simulink library "linearization"  (R2016b)
settings: Solver=VariableStepAuto  StartTime=0.0  StopTime=10.0  RelTol=1e-3
undefined symbols (not defined in the file): fsw_params
libraries: aerolibutil x2, simulink_extras x1
settings Model: Creator=bijan  LastModifiedBy=bijan

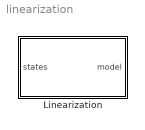
== system linearization ==
  Linearization : Subsystem

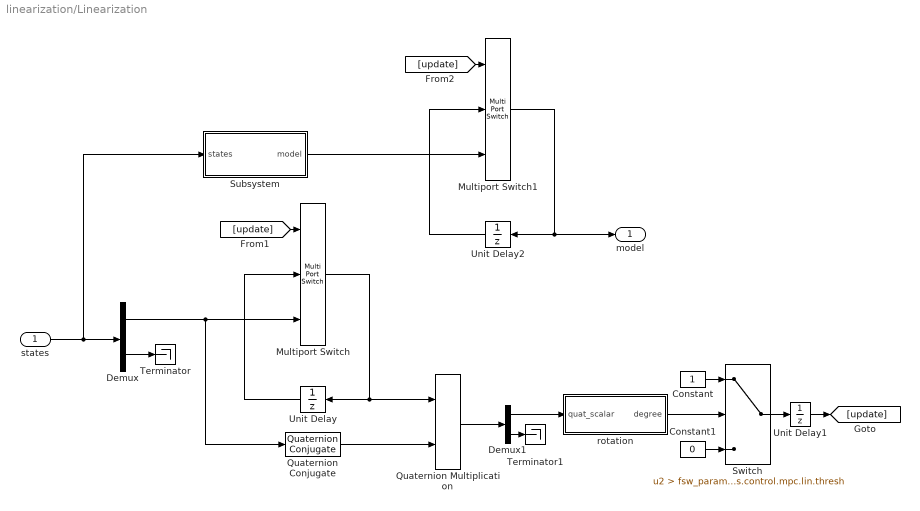
== system linearization/Linearization ==
  states : Inport
  Constant : Constant
  Constant1 : Constant  Value=0
  Demux : Demux  Outputs=[4 3]
  Demux1 : Demux  Outputs=[1 3]
  Multiport Switch : MultiPortSwitch  DataPortOrder=Zero-based contiguous  Inputs=2  DataPortIndices={0,1}
  Multiport Switch1 : MultiPortSwitch  DataPortOrder=Zero-based contiguous  Inputs=2  DataPortIndices={0,1}
  Quaternion Conjugate : aerolibutil/Quaternion Conjugate
  Quaternion Multiplication : aerolibutil/Quaternion Multiplication
  Subsystem : Subsystem
  Switch : Switch  Criteria=u2 > Threshold  Threshold=fsw_params.control.mpc.lin.thresh
  Terminator : Terminator
  Terminator1 : Terminator
  Unit Delay : UnitDelay  InitialCondition=fsw_params.control.mpc.lin.ic_quat_ud  SampleTime=-1
  Unit Delay1 : UnitDelay  InitialCondition=fsw_params.control.mpc.lin.ic_update_ud  SampleTime=-1
  Unit Delay2 : UnitDelay  InitialCondition=fsw_params.control.mpc.lin.bus_ic  SampleTime=-1
  rotation : Subsystem
  model : Outport
  wires:
  states/1 -> Subsystem/1(states), Demux/1
  Demux/2 -> Terminator/1
  Demux/1 -> Quaternion Conjugate/1, Multiport Switch/3
  Multiport Switch/1 -> Unit Delay/1, Quaternion Multiplication/1
  Unit Delay/1 -> Multiport Switch/2
  Quaternion Conjugate/1 -> Quaternion Multiplication/2
  Quaternion Multiplication/1 -> Demux1/1
  Demux1/2 -> Terminator1/1
  Demux1/1 -> rotation/1(quat_scalar)
  rotation/1(degree) -> Switch/2
  Constant/1 -> Switch/1
  Constant1/1 -> Switch/3
  Switch/1 -> Unit Delay1/1
  [update] -> Multiport Switch/1
  Unit Delay1/1 -> [update]
  Unit Delay2/1 -> Multiport Switch1/2
  Subsystem/1(model) -> Multiport Switch1/3
  Multiport Switch1/1 -> model/1, Unit Delay2/1
  [update] -> Multiport Switch1/1

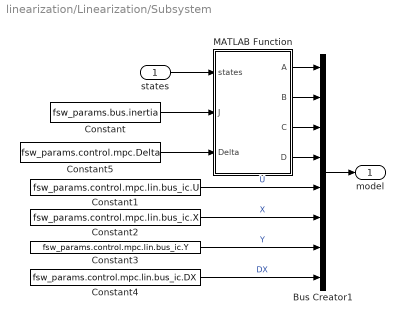
== system linearization/Linearization/Subsystem ==
  states : Inport
  Bus Creator1 : BusCreator  Inputs=8
  Constant : Constant  Value=fsw_params.bus.inertia
  Constant1 : Constant  Value=fsw_params.control.mpc.lin.bus_ic.U
  Constant2 : Constant  Value=fsw_params.control.mpc.lin.bus_ic.X
  Constant3 : Constant  Value=fsw_params.control.mpc.lin.bus_ic.Y
  Constant4 : Constant  Value=fsw_params.control.mpc.lin.bus_ic.DX
  Constant5 : Constant  Value=fsw_params.control.mpc.Delta
  MATLAB Function : MATLAB Function  TreatAsAtomicUnit=on
  model : Outport
  wires:
  MATLAB Function/1(A) -> Bus Creator1/1
  MATLAB Function/2(B) -> Bus Creator1/2
  Constant1/1 -> Bus Creator1/5  "U"
  MATLAB Function/4(D) -> Bus Creator1/4
  Constant/1 -> MATLAB Function/2(J)
  states/1 -> MATLAB Function/1(states)
  Constant3/1 -> Bus Creator1/7  "Y"
  Bus Creator1/1 -> model/1
  MATLAB Function/3(C) -> Bus Creator1/3
  Constant2/1 -> Bus Creator1/6  "X"
  Constant4/1 -> Bus Creator1/8  "DX"
  Constant5/1 -> MATLAB Function/3(Delta)

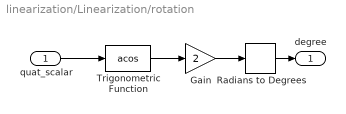
== system linearization/Linearization/rotation ==
  quat_scalar : Inport
  Gain : Gain  Gain=2
  Radians to Degrees : simulink_extras/Transformations/Radians to Degrees
  Trigonometric Function : Trigonometry  Operator=acos
  degree : Outport
  wires:
  Gain/1 -> Radians to Degrees/1
  Radians to Degrees/1 -> degree/1
  quat_scalar/1 -> Trigonometric Function/1
  Trigonometric Function/1 -> Gain/1

== matlab function linearization/Linearization/Subsystem/MATLAB Function ==
  data: states input; A output; J input; B output; C output; D output; Delta input
function [A, B, C, D] = linearization(states, J, Delta)

q = states(1:4);
w = states(5:7);

XIq     = [ q(1) -q(2)  q(3);
            q(2)  q(1) -q(4);
           -q(3)  q(4)  q(1);
           -q(2) -q(3) -q(4) ];

XIw     = [  0   -w(1)  w(2)  w(1);
            w(1)   0   -w(3)  w(2);
           -w(2)  w(3)   0    w(3);
           -w(1) -w(2) -w(3)   0  ];

AA = [ 0.5*XIw 0.5*XIq;
        zeros(3,4) zeros(3,3) ];

J_inv = inv(J);
B = Delta*[zeros(4,3); J_inv];
A = Delta*AA + eye(Nx);
C = eye(Nx);
D = zeros(7,3);
